simulink model "key_process"  (R2021a)
settings: configuration reference "f2_ctrl_config" (kept outside this file)
settings Model: DataDictionary=motor_data.sldd  Creator=Litao  LastModifiedBy=Litao
settings ConfigSetRef: SourceName=f2_ctrl_config

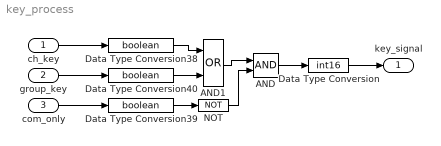
== system key_process ==
  ch_key : Inport  OutDataTypeStr=int16
  group_key : Inport  Port=2  OutDataTypeStr=int16
  com_only : Inport  Port=3  OutDataTypeStr=int16
  AND : Logic  AllPortsSameDT=off  OutDataTypeStr=boolean
  AND1 : Logic  Operator=OR  AllPortsSameDT=off  OutDataTypeStr=boolean
  Data Type Conversion : DataTypeConversion  OutDataTypeStr=int16
  Data Type Conversion38 : DataTypeConversion  OutDataTypeStr=boolean
  Data Type Conversion39 : DataTypeConversion  OutDataTypeStr=boolean
  Data Type Conversion40 : DataTypeConversion  OutDataTypeStr=boolean
  NOT : Logic  Operator=NOT  AllPortsSameDT=off  OutDataTypeStr=boolean
  key_signal : Outport  OutDataTypeStr=int16
  wires:
  Data Type Conversion39/1 -> NOT/1
  Data Type Conversion38/1 -> AND1/1
  NOT/1 -> AND/2
  com_only/1 -> Data Type Conversion39/1
  group_key/1 -> Data Type Conversion40/1
  AND1/1 -> AND/1
  AND/1 -> Data Type Conversion/1
  ch_key/1 -> Data Type Conversion38/1
  Data Type Conversion40/1 -> AND1/2
  Data Type Conversion/1 -> key_signal/1
